simulink model "ModifiedHakan"  (R2018a)
settings: Solver=VariableStepDiscrete  StartTime=0.0  StopTime=0.5  RelTol=1e-3
libraries: powerlib x21
settings Model: Creator=enes_  LastModifiedBy=enes_

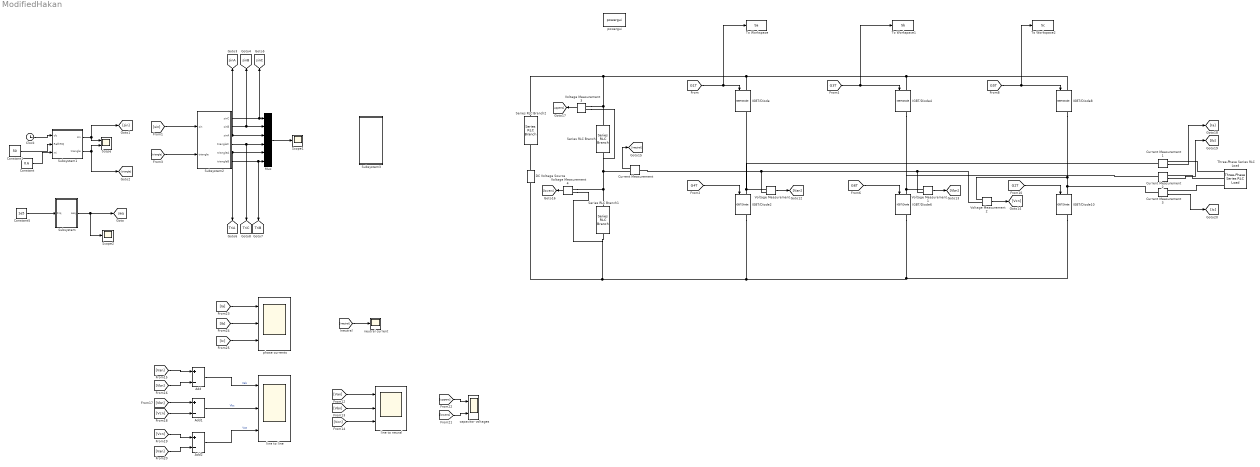
== system ModifiedHakan ==
  Add : Sum  Inputs=+-
  Add1 : Sum  Inputs=+-
  Add2 : Sum  Inputs=+-
  Clock : Clock
  Constant : Constant  Value=0.6
  Constant1 : Constant  Value=50
  Constant5 : Constant  Value=1e5
  Current Measurement{,1..3} (4 alike) : powerlib/Measurements/Current Measurement  PhasorSimulation=off  OutputType=Complex  PSBequivalent=0
  DC Voltage Source : powerlib/Electrical Sources/DC Voltage Source  Amplitude=540  Measurements=None
  IGBT/Diode{,2,4,6,8,10} (6 alike) : powerlib/Power Electronics/IGBT//Diode  Ron=1e-3  Rs=1e5  Cs=inf  Measurements=on
  Mux : Mux  Inputs=6
  Scope : Scope  NumInputPorts=2
  Scope1 : Scope
  Scope2 : Scope
  Series RLC Branch : powerlib/Elements/Series RLC Branch  LConnTagsString=__new0  RConnTagsString=__new0  BranchType=C  Resistance=1  Inductance=1e-3  SetiL0=off  InitialCurrent=0  Capacitance=1000e-6  Setx0=off  InitialVoltage=0  Measurements=None
  Series RLC Branch1 : powerlib/Elements/Series RLC Branch  LConnTagsString=__new0  RConnTagsString=__new0  BranchType=C  Resistance=1  Inductance=1e-3  SetiL0=off  InitialCurrent=0  Capacitance=1000e-6  Setx0=off  InitialVoltage=0  Measurements=None
  Series RLC Branch2 : powerlib/Elements/Series RLC Branch  LConnTagsString=__new0  RConnTagsString=__new0  BranchType=R  Resistance=1  Inductance=1e-3  SetiL0=off  InitialCurrent=0  Capacitance=1000e-6  Setx0=off  InitialVoltage=0  Measurements=None
  Subsystem : Subsystem
  Subsystem1 : Subsystem
  Subsystem2 : Subsystem
  Subsystem3 : Subsystem
  Three-Phase Series RLC Load : powerlib/Elements/Three-Phase Series RLC Load  LConnTagsString=A|B|C  Configuration=Y (floating)  NominalVoltage=1000  Vabc=[1e3 1e3 1e3]  Vabcp=[1e3 1e3 1e3]  NominalFrequency=50  UnbalancedPower=off  ActivePower=8000  InductivePower=3870  CapacitivePower=0  Pabc=[10e3 9e3 11e3]  QLabc=[100 90 110]  QCabc=[100 90 110]  Pabcp=[10e3 9e3 11e3]  QLabcp=[100 90 110]  QCabcp=[100 90 110]  Measurements=None  LoadType=constant Z
  To Workspace : ToWorkspace  VariableName=Sa  SaveFormat=Timeseries  SampleTime=-1
  To Workspace1 : ToWorkspace  VariableName=Sb  SaveFormat=Timeseries  SampleTime=-1
  To Workspace2 : ToWorkspace  VariableName=Sc  SaveFormat=Timeseries  SampleTime=-1
  Voltage Measurement{,1..4} (5 alike) : powerlib/Measurements/Voltage Measurement  PhasorSimulation=off  OutputType=Complex  PSBequivalent=0
  capacitor voltages : Scope  NumInputPorts=2
  line to line : Scope  NumInputPorts=3
  line to neural : Scope  NumInputPorts=3
  neutral current : Scope
  phase currents : Scope  NumInputPorts=3
  powergui : powerlib/powergui  Priority=1  SimulationMode=Discrete  SampleTime=1e-7  frequency=60  Iterations=50  frequencyindice=0  Pbase=100e6  ErrMax=1e-4  UnitsV=kV  UnitsW=MW  buscounter=0  FunctionMessages=off  echomessages=off  EnableUseOfTLC=off  CurrentSourceSwitches=off  DisableSnubberDevices=off  DisableRonSwitches=off  DisableVfSwitches=off  DisplayEquations=off  SolverType=Tustin/Backward Euler (TBE)  Interpol=off  ExternalGateDelay=off  methode=off  Ts=100  x0status=blocks  SPID=off  SwTol=0  HookPort=off  RestoreLinks=warning  ResistiveCurrentMeasurement=off  Frange=[0:2:500]  Ylog=off  Xlog=on  ShowGrid=off  save=off  variable=ZData  structure=linetoline  ZoomFFT=off  StartTime=0.0  cycles=2  DisplayStyle=1  fundamental=50  FreqAxis=off  MaxFrequency=5000  frequencyindicesteady=1  RmsSteady=1  display=off
  tag scope: TriA=global, TriB=global, TriC=global, seq=global, sinA=global, sinB=global, sinC=global
  wires:
  [Vcn] -> line to neural/3
  [G2T] -> IGBT/Diode10/1
  [G1T] -> To Workspace/1, IGBT/Diode/1
  [Vbn] -> line to neural/2
  [G6T] -> IGBT/Diode6/1
  Voltage Measurement1/1 -> [Vbn]
  [G5T] -> To Workspace2/1, IGBT/Diode8/1
  [Ic] -> phase currents/3
  Voltage Measurement/1 -> [Van]
  [G4T] -> IGBT/Diode2/1
  [Van] -> Add/1
  Add2/1 -> line to line/3  "Vca"
  [Van] -> Add2/2
  Add1/1 -> line to line/2  "Vbc"
  [Vcn] -> Add2/1
  [Van] -> line to neural/1
  [Vbn] -> Add/2
  [Ineutral] -> neutral current/1
  [upperc] -> capacitor voltages/1
  Add/1 -> line to line/1  "Vab"
  [Ib] -> phase currents/2
  Current Measurement2/1 -> [Ib]
  [Vcn] -> Add1/2
  [lowerc] -> capacitor voltages/2
  [Ia] -> phase currents/1
  [Vbn] -> Add1/1
  Voltage Measurement4/1 -> [lowerc]
  Voltage Measurement2/1 -> [Vcn]
  Current Measurement/1 -> [Ineutral]
  Voltage Measurement3/1 -> [upperc]
  Current Measurement3/1 -> [Ic]
  Current Measurement1/1 -> [Ia]
  Subsystem2/2(sinB) -> Mux/2, [sinB]
  Mux/1 -> Scope1/1
  [triangle] -> Subsystem2/2(triangle)
  [sin] -> Subsystem2/1(sin)
  Subsystem2/1(sinC) -> [sinC], Mux/1
  Constant/1 -> Subsystem1/3(mi)
  Subsystem2/4(triangleC) -> [TriC], Mux/4
  Subsystem2/5(triangleA) -> Mux/5, [TriA]
  Clock/1 -> Subsystem1/1(clc)
  Subsystem1/2(triangle) -> [triangle], Scope/2
  Constant1/1 -> Subsystem1/2(RefFRQ)
  Subsystem1/1(sin) -> [sin], Scope/1
  Subsystem/1("seq ") -> Scope2/1, [seq]
  Constant5/1 -> Subsystem/1(Frq)
  Subsystem2/6(triangleB) -> [TriB], Mux/6
  Subsystem2/3(sinA) -> Mux/3, [sinA]
  [G3T] -> To Workspace1/1, IGBT/Diode4/1
  connections:
  Voltage Measurement1/LConn1 -- IGBT/Diode6/LConn1 -- Current Measurement2/LConn1 -- IGBT/Diode4/RConn1
  IGBT/Diode6/RConn1 -- IGBT/Diode10/RConn1 -- IGBT/Diode2/RConn1 -- DC Voltage Source/LConn1 -- Voltage Measurement4/LConn2 -- Series RLC Branch1/RConn1
  IGBT/Diode8/LConn1 -- Series RLC Branch/LConn1 -- Voltage Measurement3/LConn1 -- Series RLC Branch2/LConn1 -- IGBT/Diode/LConn1 -- IGBT/Diode4/LConn1
  Voltage Measurement1/LConn2 -- Voltage Measurement2/LConn2 -- Current Measurement/LConn1 -- Voltage Measurement/LConn2
  Voltage Measurement/LConn1 -- IGBT/Diode2/LConn1 -- Current Measurement1/LConn1 -- IGBT/Diode/RConn1
  Voltage Measurement4/LConn1 -- Voltage Measurement3/LConn2 -- Series RLC Branch/RConn1 -- Current Measurement/RConn1 -- Series RLC Branch1/LConn1
  IGBT/Diode8/RConn1 -- Voltage Measurement2/LConn1 -- IGBT/Diode10/LConn1 -- Current Measurement3/LConn1
  Three-Phase Series RLC Load/LConn1 -- Current Measurement1/RConn1
  DC Voltage Source/RConn1 -- Series RLC Branch2/RConn1
  Three-Phase Series RLC Load/LConn2 -- Current Measurement2/RConn1
  Three-Phase Series RLC Load/LConn3 -- Current Measurement3/RConn1

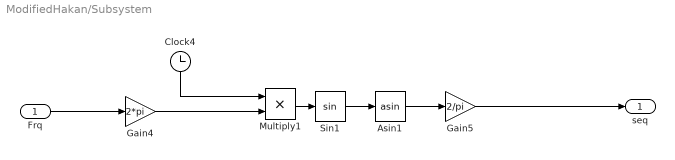
== system ModifiedHakan/Subsystem ==
  Frq : Inport
  Asin1 : Trigonometry  Operator=asin
  Clock4 : Clock
  Gain4 : Gain  Gain=2*pi
  Gain5 : Gain  Gain=2/pi
  Multiply1 : Product
  Sin1 : Trigonometry
  "seq " : Outport
  wires:
  Frq/1 -> Gain4/1
  Asin1/1 -> Gain5/1
  Gain5/1 -> "seq "/1
  Multiply1/1 -> Sin1/1
  Sin1/1 -> Asin1/1
  Gain4/1 -> Multiply1/2
  Clock4/1 -> Multiply1/1

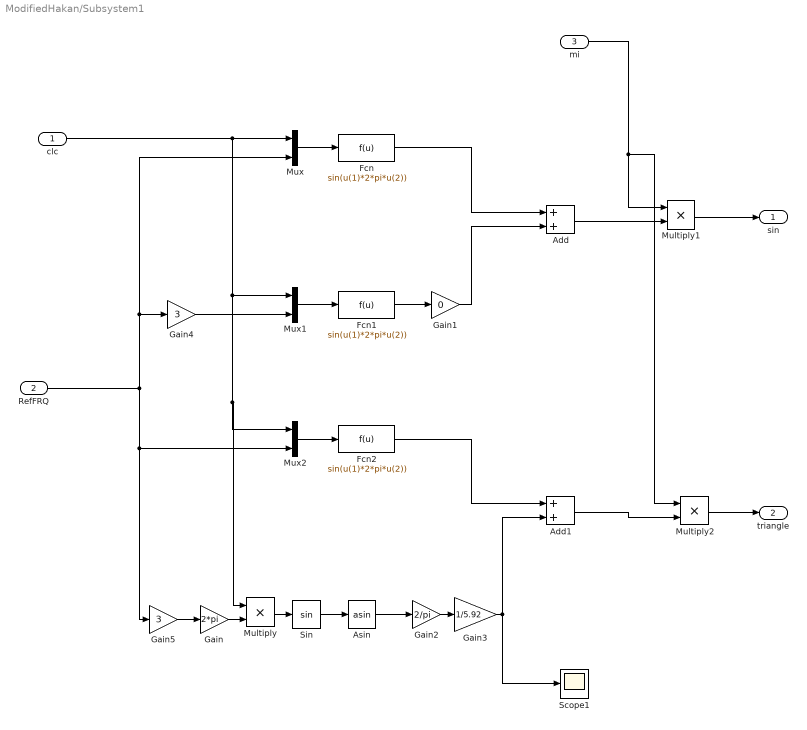
== system ModifiedHakan/Subsystem1 ==
  clc : Inport
  RefFRQ : Inport  Port=2
  mi : Inport  Port=3
  Add : Sum
  Add1 : Sum
  Asin : Trigonometry  Operator=asin
  Fcn : Fcn  Expr=sin(u(1)*2*pi*u(2))
  Fcn1 : Fcn  Expr=sin(u(1)*2*pi*u(2))
  Fcn2 : Fcn  Expr=sin(u(1)*2*pi*u(2))
  Gain : Gain  Gain=2*pi
  Gain1 : Gain  Gain=0
  Gain2 : Gain  Gain=2/pi
  Gain3 : Gain  Gain=1/5.92
  Gain4 : Gain  Gain=3
  Gain5 : Gain  Gain=3
  Multiply : Product
  Multiply1 : Product
  Multiply2 : Product
  Mux : Mux  Inputs=2
  Mux1 : Mux  Inputs=2
  Mux2 : Mux  Inputs=2
  Scope1 : Scope
  Sin : Trigonometry
  sin : Outport
  triangle : Outport  Port=2
  wires:
  Fcn1/1 -> Gain1/1
  Mux2/1 -> Fcn2/1
  Mux1/1 -> Fcn1/1
  Mux/1 -> Fcn/1
  Asin/1 -> Gain2/1
  clc/1 -> Multiply/1, Mux2/1, Mux1/1, Mux/1
  Fcn/1 -> Add/1
  Sin/1 -> Asin/1
  Gain/1 -> Multiply/2
  Gain2/1 -> Gain3/1
  Gain1/1 -> Add/2
  Multiply/1 -> Sin/1
  Gain4/1 -> Mux1/2
  Fcn2/1 -> Add1/1
  Gain3/1 -> Scope1/1, Add1/2
  RefFRQ/1 -> Mux/2, Gain4/1, Gain5/1, Mux2/2
  Gain5/1 -> Gain/1
  Add/1 -> Multiply1/2
  Multiply1/1 -> sin/1
  Add1/1 -> Multiply2/2
  Multiply2/1 -> triangle/1
  mi/1 -> Multiply2/1, Multiply1/1

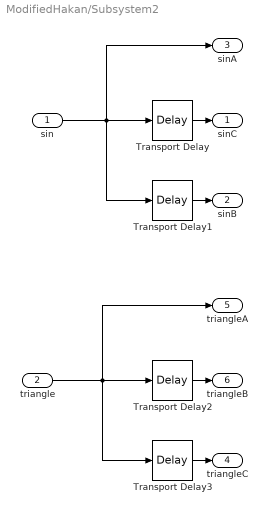
== system ModifiedHakan/Subsystem2 ==
  sin : Inport
  triangle : Inport  Port=2
  Transport Delay : TransportDelay  DelayTime=(1/150)
  Transport Delay1 : TransportDelay  DelayTime=2/150
  Transport Delay2 : TransportDelay  DelayTime=(1/150)
  Transport Delay3 : TransportDelay  DelayTime=2/150
  sinC : Outport
  sinB : Outport  Port=2
  sinA : Outport  Port=3
  triangleC : Outport  Port=4
  triangleA : Outport  Port=5
  triangleB : Outport  Port=6
  wires:
  Transport Delay1/1 -> sinB/1
  sin/1 -> sinA/1, Transport Delay1/1, Transport Delay/1
  Transport Delay2/1 -> triangleB/1
  triangle/1 -> triangleA/1, Transport Delay3/1, Transport Delay2/1
  Transport Delay3/1 -> triangleC/1
  Transport Delay/1 -> sinC/1

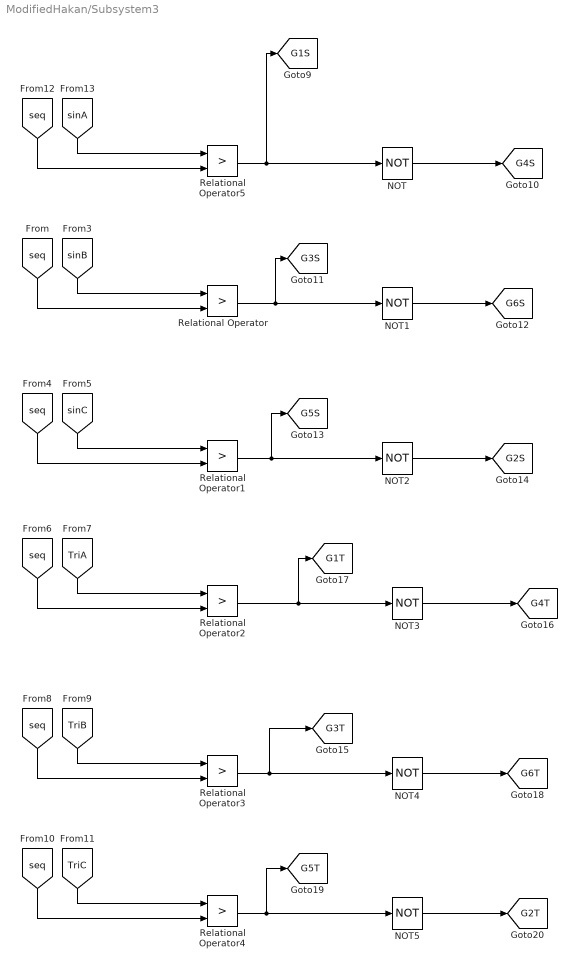
== system ModifiedHakan/Subsystem3 ==
  NOT{,1..5} (6 alike) : Logic  Operator=NOT  AllPortsSameDT=off  OutDataTypeStr=boolean
  Relational Operator{,1..5} (6 alike) : RelationalOperator  Operator=>  OutDataTypeStr=boolean  RndMeth=Simplest
  tag scope: G1S=global, G1T=global, G2S=global, G2T=global, G3S=global, G3T=global, G4S=global, G4T=global, G5S=global, G5T=global, G6S=global, G6T=global
  wires:
  [sinC] -> Relational Operator1/1
  [TriB] -> Relational Operator3/1
  NOT3/1 -> [G4T]
  Relational Operator/1 -> [G3S], NOT1/1
  [seq] -> Relational Operator4/2
  [sinB] -> Relational Operator/1
  [TriC] -> Relational Operator4/1
  Relational Operator5/1 -> [G1S], NOT/1
  [seq] -> Relational Operator3/2
  NOT4/1 -> [G6T]
  Relational Operator3/1 -> NOT4/1, [G3T]
  [sinA] -> Relational Operator5/1
  Relational Operator1/1 -> [G5S], NOT2/1
  Relational Operator2/1 -> [G1T], NOT3/1
  [seq] -> Relational Operator5/2
  [seq] -> Relational Operator/2
  Relational Operator4/1 -> [G5T], NOT5/1
  NOT5/1 -> [G2T]
  NOT/1 -> [G4S]
  [seq] -> Relational Operator2/2
  [TriA] -> Relational Operator2/1
  [seq] -> Relational Operator1/2
  NOT1/1 -> [G6S]
  NOT2/1 -> [G2S]
